simulink model "Zadatak_31"  (R2020b)
settings: Solver=VariableStepAuto  StartTime=0.0  StopTime=1  RelTol=1e-3
values from neighbouring files (symbols this model uses):
  k = k+1    (= 2)    [Zadatak_22.m]    (also in Zadatak_23.m)
undefined symbols (not defined in the file or in its folder): Kg, q, Rp, Rs
libraries: simulink x2
settings Model: Creator=user  LastModifiedBy=user

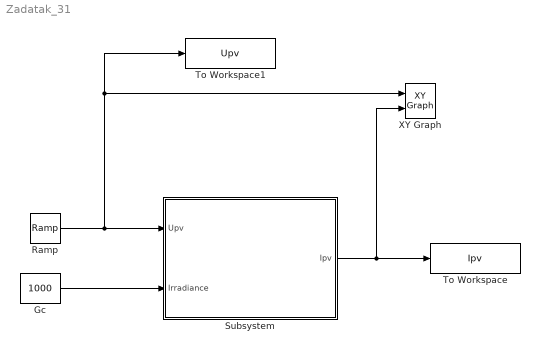
== system Zadatak_31 ==
  Gc : Constant  Value=1000
  Ramp : simulink/Sources/Ramp  slope=0.7  start=0  InitialOutput=0
  Subsystem : Subsystem
  To Workspace : ToWorkspace  VariableName=Ipv  SaveFormat=Timeseries  SampleTime=-1
  To Workspace1 : ToWorkspace  VariableName=Upv  SampleTime=-1
  XY Graph : simulink/Sinks/XY Graph  xmin=0  xmax=0.6  ymin=0  ymax=1.2  st=-1
  wires:
  Subsystem/1(Ipv) -> XY Graph/2, To Workspace/1
  Ramp/1 -> To Workspace1/1, XY Graph/1, Subsystem/1(Upv)
  Gc/1 -> Subsystem/2(Irradiance)

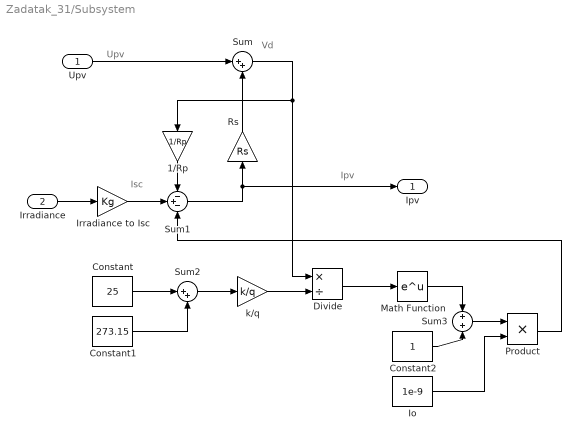
== system Zadatak_31/Subsystem ==
  note: Ipv
  note: Isc
  note: Vd
  note: Upv
  Upv : Inport
  Irradiance : Inport  Port=2
  1/Rp : Gain  Gain=1/Rp
  Constant : Constant  Value=25
  Constant1 : Constant  Value=273.15
  Constant2 : Constant
  Divide : Product  Inputs=*/
  Io : Constant  Value=1e-9
  Irradiance to Isc : Gain  Gain=Kg
  Math Function : Math  SaturateOnIntegerOverflow=on
  Product : Product
  Rs : Gain  Gain=Rs
  Sum : Sum  Inputs=|++
  Sum1 : Sum  Inputs=-+-
  Sum2 : Sum  Inputs=|++
  Sum3 : Sum
  k/q : Gain  Gain=k/q
  Ipv : Outport
  wires:
  Upv/1 -> Sum/1
  Divide/1 -> Math Function/1
  Sum/1 -> 1/Rp/1, Divide/1
  k/q/1 -> Divide/2
  Sum1/1 -> Rs/1, Ipv/1
  Irradiance/1 -> Irradiance to Isc/1
  1/Rp/1 -> Sum1/1
  Irradiance to Isc/1 -> Sum1/2
  Rs/1 -> Sum/2
  Constant/1 -> Sum2/1
  Constant1/1 -> Sum2/2
  Sum2/1 -> k/q/1
  Math Function/1 -> Sum3/1
  Constant2/1 -> Sum3/2
  Sum3/1 -> Product/1
  Io/1 -> Product/2
  Product/1 -> Sum1/3
